simulink subsystem "PowerSystemRef"  (R2024b)
settings: Solver=VariableStepAuto  StartTime=0.0  StopTime=10.0  RelTol=1e-3
undefined symbols (not defined in the file): ess, geom, mot, mot2, mot3, mot4, propel, propel2, propel3, propel4, pxf_diagram_options, SimIn, tc, tc2, tc3, tc4
libraries: simulink x10, slpidlib x5
(part 6 of 10)

== system PowerSystemRef/propel/plant/propel_plant_uas/Thrust_Generated ==
  env_plant_density_simu : Inport
  propel_plant_speed_simu : Inport  Port=2
  Mux5 : Mux  Inputs=3
  RPS2T : Fcn  Expr=u(2) * u(3) * propel.plant.init.propD^4 * u(1)^2
  propel_plant_init_CP_CT_map : Subsystem  mask{x=propel.plant.init.CP_CT_map(:,1)/60, map=propel.plant.init.CP_CT_map(:,2)}
  propel_plant_thrust_simu : Outport  VectorParamsAs1DForOutWhenUnconnected=off
  propel_plant_CT_simu : Outport  Port=2  VectorParamsAs1DForOutWhenUnconnected=off
  wires:
  propel_plant_init_CP_CT_map/1(output) -> propel_plant_CT_simu/1, Mux5/2
  env_plant_density_simu/1 -> Mux5/3
  propel_plant_speed_simu/1 -> propel_plant_init_CP_CT_map/1(input x), Mux5/1
  Mux5/1 -> RPS2T/1
  RPS2T/1 -> propel_plant_thrust_simu/1

== system PowerSystemRef/propel/plant/propel_plant_uas/Total_Moment ==
  propel_plant_thrust_simu : Inport
  propel_plant_restq_simu : Inport  Port=2
  Gain : Gain  Gain=-propel.plant.init.rotationdir
  Gain1 : Gain  Gain=propel.plant.init.thrustdir
  Moment_due_to_eng_position : Subsystem
  Sum2 : Sum  Inputs=|+-  SaturateOnIntegerOverflow=on
  Sum4 : Sum  SaturateOnIntegerOverflow=on
  geom.init.CG : Constant  Value=SimIn.Model.cm_b
  propel.plant.init.pos : Constant  Value=propel.plant.init.pos
  accmoment_plant_totmoment_simu : Outport  VectorParamsAs1DForOutWhenUnconnected=off
  wires:
  propel_plant_restq_simu/1 -> Gain/1
  Gain1/1 -> Moment_due_to_eng_position/2(Vec 2)
  Gain/1 -> Sum4/2
  Sum2/1 -> Moment_due_to_eng_position/1(Vec 1)
  Sum4/1 -> accmoment_plant_totmoment_simu/1  "accmoment_plant_totmoment_simu"
  propel.plant.init.pos/1 -> Sum2/1
  geom.init.CG/1 -> Sum2/2
  propel_plant_thrust_simu/1 -> Gain1/1
  Moment_due_to_eng_position/1(X Prod) -> Sum4/1

== system PowerSystemRef/tc/plant/tc_plant_map_trqloss_funTW/Inertia calculation ==
  inertia in : Inport
  Sum3 : Sum  Inputs=|++  InputSameDT=on  SaturateOnIntegerOverflow=on  OutDataTypeStr=Inherit: Same as first input
  tc inertia : Constant  Value=tc.plant.init.inertia
  tc.plant.init.ratio : Gain  Gain=tc.plant.init.ratio
  "tc.plant.init.ratio " : Gain  Gain=tc.plant.init.ratio
  inertia out : Outport
  wires:
  "tc.plant.init.ratio "/1 -> tc.plant.init.ratio/1
  inertia in/1 -> "tc.plant.init.ratio "/1
  tc.plant.init.ratio/1 -> Sum3/1
  tc inertia/1 -> Sum3/2
  Sum3/1 -> inertia out/1

== system PowerSystemRef/tc/plant/tc_plant_map_trqloss_funTW/Speed calculation ==
  spd out : Inport
  tc.plant.init.ratio : Gain  Gain=tc.plant.init.ratio
  spd in : Outport
  wires:
  spd out/1 -> tc.plant.init.ratio/1
  tc.plant.init.ratio/1 -> spd in/1

== system PowerSystemRef/tc/plant/tc_plant_map_trqloss_funTW/Torque calculation ==
  spd in : Inport
  trq in : Inport  Port=2
  Abs : Abs
  Abs1 : Abs
  Blending (state dependent) : Subsystem  mask(State dependent blending){xl=-tc.plant.init.spd_thresh, yl=-1, xc=0, yc=0, xr=tc.plant.init.spd_thresh, yr=1}
      mask prompts: xl "Left point (x):"; yl "Left point (y):"; xc "Center point (x):"; yc "Center point (y):"; xr "Right point (x):"; yr "Right point (y):"
      mask help: This block implements state dependent smoothing/blending. IMPORTANT: See help menu.
      mask Help: The output equals the product of the first input and a "hat" function defined by the three points specified in the dialog box.  The second input forms the argument to the hat function.\n\nIMPORTANT: A divide by zero error will result if first coordinates of the three points specified for the hat function are NOT distinct.
      mask Display: plot([-1 1 3 6 8], [1.5 1.5 0.5 4.0 4.0])
  Sum2 : Sum  Inputs=|+-  InputSameDT=on  SaturateOnIntegerOverflow=on  OutDataTypeStr=Inherit: Same as first input
  tc.plant.init.ratio : Gain  Gain=tc.plant.init.ratio
  trq losses : Subsystem  mask(Lookup Table (2-D)){x=tc.plant.init.trq_loss.idx1_trq, y=tc.plant.init.trq_loss.idx2_spd, t=tc.plant.init.trq_loss.map}
      mask prompts: x "Row:"; y "Column:"; t "Table:"
      mask help: Performs 2-D linear interpolation of input values using the specified input/output table. Extrapolation is performed outside the table boundaries.
      mask init:
      | [r,c]=size(t);
      | xt=reshape(x,prod(size(x)),1);
      | xi=xt(:,ones(1,c));
      | minx=min(x); maxx=max(x);
      | mint=min(min(t)); maxt=max(max(t));
      mask Display: plot(xi,t,[minx maxx],[mint mint],[minx minx],[mint maxt])
  trq out : Outport
  wires:
  tc.plant.init.ratio/1 -> trq out/1
  Sum2/1 -> tc.plant.init.ratio/1
  trq in/1 -> Sum2/1, Abs/1
  spd in/1 -> Blending (state dependent)/2(Control (state)), Abs1/1
  Blending (state dependent)/1(Output) -> Sum2/2
  trq losses/1(Out1) -> Blending (state dependent)/1(Input)
  Abs1/1 -> trq losses/2(Cols)
  Abs/1 -> trq losses/1(Rows)

== system PowerSystemRef/ess (battery)/ctrl/ess_ctrl_pngv_map_anl_PI_cstr/PI controller for maximal charge power and current1/PI Ratio Calculator (curr)  ==
  note: %deviation
  ess curr : Inport
  curr max cont : Inport  Port=2
  Add1 : Sum  Inputs=-+
  Integrator1 : Integrator  InitialCondition=ess.plant.init.ul_curr_chg  LimitOutput=on  UpperSaturationLimit=ess.plant.init.ul_curr_chg  LowerSaturationLimit=ess.plant.init.ll_curr_chg
  Ki_curr : Gain  Gain=ess.plant.init.Ki_curr_chg  SaturateOnIntegerOverflow=on  OutDataTypeStr=Inherit: Same as input  ParamDataTypeStr=Inherit: Same as input
  Saturation1 : Saturate  UpperLimit=1  LowerLimit=0
  non-zero division1 : Subsystem
      mask Display: disp('divider')
  Current ratio : Outport
  wires:
  Add1/1 -> non-zero division1/1(In1)
  non-zero division1/1(Out1) -> Ki_curr/1
  Ki_curr/1 -> Integrator1/1
  Integrator1/1 -> Saturation1/1
  ess curr/1 -> Add1/1
  Saturation1/1 -> Current ratio/1
  curr max cont/1 -> Add1/2, non-zero division1/2(In2)

== system PowerSystemRef/ess (battery)/ctrl/ess_ctrl_pngv_map_anl_PI_cstr/PI controller for maximal charge power and current1/PI Ratio Calculator (curr) 1 ==
  note: %deviation
  ess pwr : Inport
  pwr max cont : Inport  Port=2
  Add1 : Sum  Inputs=-+
  Integrator1 : Integrator  InitialCondition=ess.plant.init.ul_curr_dis  LimitOutput=on  UpperSaturationLimit=ess.plant.init.ul_curr_dis  LowerSaturationLimit=ess.plant.init.ll_curr_dis
  Ki_pwr : Gain  Gain=ess.plant.init.Ki_pwr_chg  SaturateOnIntegerOverflow=on  OutDataTypeStr=Inherit: Same as input  ParamDataTypeStr=Inherit: Same as input
  Saturation1 : Saturate  UpperLimit=1  LowerLimit=0
  non-zero division1 : Subsystem
      mask Display: disp('divider')
  pwr ratio : Outport
  wires:
  Add1/1 -> non-zero division1/1(In1)
  non-zero division1/1(Out1) -> Ki_pwr/1
  Ki_pwr/1 -> Integrator1/1
  Integrator1/1 -> Saturation1/1
  ess pwr/1 -> Add1/1
  Saturation1/1 -> pwr ratio/1
  pwr max cont/1 -> Add1/2, non-zero division1/2(In2)

== system PowerSystemRef/ess (battery)/ctrl/ess_ctrl_pngv_map_anl_PI_cstr/PI controller for maximal discharge power and current1/PI Ratio Calculator (curr)  ==
  note: %deviation
  ess curr : Inport
  curr max cont : Inport  Port=2
  Add1 : Sum  Inputs=-+
  Integrator1 : Integrator  InitialCondition=ess.plant.init.ul_curr_dis  LimitOutput=on  UpperSaturationLimit=ess.plant.init.ul_curr_dis  LowerSaturationLimit=ess.plant.init.ll_curr_dis
  Ki_curr : Gain  Gain=ess.plant.init.Ki_curr_dis  SaturateOnIntegerOverflow=on  OutDataTypeStr=Inherit: Same as input  ParamDataTypeStr=Inherit: Same as input
  Saturation1 : Saturate  UpperLimit=1  LowerLimit=0
  non-zero division1 : Subsystem
      mask Display: disp('divider')
  Current ratio : Outport
  wires:
  curr max cont/1 -> non-zero division1/2(In2), Add1/2
  Saturation1/1 -> Current ratio/1
  ess curr/1 -> Add1/1
  Integrator1/1 -> Saturation1/1
  Ki_curr/1 -> Integrator1/1
  non-zero division1/1(Out1) -> Ki_curr/1
  Add1/1 -> non-zero division1/1(In1)

== system PowerSystemRef/ess (battery)/ctrl/ess_ctrl_pngv_map_anl_PI_cstr/PI controller for maximal discharge power and current1/PI Ratio Calculator (curr) 1 ==
  note: %deviation
  ess pwr : Inport
  pwr max cont : Inport  Port=2
  Add1 : Sum  Inputs=-+
  Integrator1 : Integrator  InitialCondition=ess.plant.init.ul_curr_dis  LimitOutput=on  UpperSaturationLimit=ess.plant.init.ul_curr_dis  LowerSaturationLimit=ess.plant.init.ll_curr_dis
  Ki_pwr : Gain  Gain=ess.plant.init.Ki_pwr_dis  SaturateOnIntegerOverflow=on  OutDataTypeStr=Inherit: Same as input  ParamDataTypeStr=Inherit: Same as input
  Saturation1 : Saturate  UpperLimit=1  LowerLimit=0
  non-zero division1 : Subsystem
      mask Display: disp('divider')
  pwr ratio : Outport
  wires:
  Add1/1 -> non-zero division1/1(In1)
  non-zero division1/1(Out1) -> Ki_pwr/1
  Ki_pwr/1 -> Integrator1/1
  Integrator1/1 -> Saturation1/1
  ess pwr/1 -> Add1/1
  Saturation1/1 -> pwr ratio/1
  pwr max cont/1 -> Add1/2, non-zero division1/2(In2)

== system PowerSystemRef/ess (battery)/plant/ess_plant_pngv_map_anl_PI_cstr/ess_cell/current polarization ==
  ess soc : Inport
  ess curr : Inport  Port=2
  Integrator : Integrator
  Product1 : Product  Inputs=*/  InputSameDT=on  SaturateOnIntegerOverflow=on  OutDataTypeStr=Inherit: Same as first input
  Sum1 : Sum  Inputs=+-  InputSameDT=on  SaturateOnIntegerOverflow=on  OutDataTypeStr=Inherit: Same as first input
  Time Constant : Lookup  InputValues=ess.plant.init.tau1.idx1_soc  Table=ess.plant.init.tau1.map
  ess_cell_curr_polar1 : Outport
  wires:
  Time Constant/1 -> Product1/2
  Product1/1 -> Integrator/1
  ess soc/1 -> Time Constant/1
  ess curr/1 -> Sum1/1
  Sum1/1 -> Product1/1
  Integrator/1 -> Sum1/2, ess_cell_curr_polar1/1

== system PowerSystemRef/ess (battery)/plant/ess_plant_pngv_map_anl_PI_cstr/ess_cell/current polarization1 ==
  ess soc : Inport
  ess curr : Inport  Port=2
  Integrator : Integrator
  Product1 : Product  Inputs=*/  InputSameDT=on  SaturateOnIntegerOverflow=on  OutDataTypeStr=Inherit: Same as first input
  Sum1 : Sum  Inputs=+-  InputSameDT=on  SaturateOnIntegerOverflow=on  OutDataTypeStr=Inherit: Same as first input
  Time Constant : Lookup  InputValues=ess.plant.init.tau2.idx1_soc  Table=ess.plant.init.tau2.map
  ess_cell_curr_polar2 : Outport
  wires:
  Integrator/1 -> ess_cell_curr_polar2/1, Sum1/2
  Sum1/1 -> Product1/1
  ess curr/1 -> Sum1/1
  ess soc/1 -> Time Constant/1
  Product1/1 -> Integrator/1
  Time Constant/1 -> Product1/2

== system PowerSystemRef/ess (battery)/plant/ess_plant_pngv_map_anl_PI_cstr/ess_cell/ess_soc_calculation ==
  cell_curr : Inport
  (sec->hrs) : Gain  Gain=1/3600  SaturateOnIntegerOverflow=on  OutDataTypeStr=Inherit: Same as input  ParamDataTypeStr=Inherit: Same as input
  (sec->hrs)1 : Gain  Gain=-1  SaturateOnIntegerOverflow=on  OutDataTypeStr=Inherit: Same as input  ParamDataTypeStr=Inherit: Same as input
  0 <= SOC <= 1 : Saturate  UpperLimit=1  LowerLimit=0
  1\ess.plant.init.cap : Gain  Gain=1/ess.plant.init.cap  SaturateOnIntegerOverflow=on  OutDataTypeStr=Inherit: Same as input  ParamDataTypeStr=Inherit: Same as input
  Integrator : Integrator  InitialCondition=ess.plant.init.soc_init
  ess_soc : Outport
  wires:
  (sec->hrs)/1 -> 1\ess.plant.init.cap/1
  0 <= SOC <= 1/1 -> ess_soc/1
  Integrator/1 -> 0 <= SOC <= 1/1
  (sec->hrs)1/1 -> Integrator/1
  1\ess.plant.init.cap/1 -> (sec->hrs)1/1
  cell_curr/1 -> (sec->hrs)/1

== system PowerSystemRef/ess (battery)/plant/ess_plant_pngv_map_anl_PI_cstr/ess_cell/voltage calculation ==
  absolute SOC : Inport
  ess_cell_curr : Inport  Port=2
  ess_cell_curr_pol1 : Inport  Port=3
  ess_cell_curr_plo2 : Inport  Port=4
  Ohmic resist : Lookup  InputValues=ess.plant.init.rint.idx1_soc  Table=ess.plant.init.rint.map
  "Polarization resist 2 " : Lookup  InputValues=ess.plant.init.rpol2.idx1_soc  Table=ess.plant.init.rpol2.map
  Polarization resist2 : Lookup  InputValues=ess.plant.init.rpol1.idx1_soc  Table=ess.plant.init.rpol1.map
  Product1 : Product  InputSameDT=on  SaturateOnIntegerOverflow=on  OutDataTypeStr=Inherit: Same as first input
  Product2 : Product  InputSameDT=on  SaturateOnIntegerOverflow=on  OutDataTypeStr=Inherit: Same as first input
  Product3 : Product  InputSameDT=on  SaturateOnIntegerOverflow=on  OutDataTypeStr=Inherit: Same as first input
  Saturation : Saturate  UpperLimit=inf  LowerLimit=ess.plant.init.volt_min_burst
  Sum2 : Sum  Inputs=+---  InputSameDT=on  SaturateOnIntegerOverflow=on  OutDataTypeStr=Inherit: Same as first input
  Voc : Lookup  InputValues=ess.plant.init.voc.idx1_soc  Table=ess.plant.init.voc.map
  ess_cell_volt : Outport
  ess_cell_voc : Outport  Port=2
  ess_cell_rint : Outport  Port=3
  ess_cell_rpol1 : Outport  Port=4
  ess_cell_rpol2 : Outport  Port=5
  wires:
  Saturation/1 -> ess_cell_volt/1
  "Polarization resist 2 "/1 -> ess_cell_rpol2/1, Product3/2  "ess_rpol2_simu"
  ess_cell_curr_plo2/1 -> Product3/1
  Product3/1 -> Sum2/4
  Product2/1 -> Sum2/3
  Polarization resist2/1 -> ess_cell_rpol1/1, Product2/2  "ess_rpol1_simu"
  ess_cell_curr_pol1/1 -> Product2/1
  Product1/1 -> Sum2/2
  absolute SOC/1 -> Voc/1, Ohmic resist/1, Polarization resist2/1, "Polarization resist 2 "/1
  Voc/1 -> ess_cell_voc/1, Sum2/1  "ess_voc_simu"
  ess_cell_curr/1 -> Product1/1
  Ohmic resist/1 -> ess_cell_rint/1, Product1/2  "ess_rint_simu"
  Sum2/1 -> Saturation/1

== system PowerSystemRef/mot/ctrl/cmd/mot_ctrl_cmd_map_Pelec_funTW_volt_in/Subsystem2 ==
  In1 : Inport
  In2 : Inport  Port=2
  Fcn : Fcn  Expr=u[1]/(u[2]+eps)*(u[2]!=0)
  Mux : Mux  Inputs=2
  Out1 : Outport
  wires:
  In2/1 -> Mux/2
  Fcn/1 -> Out1/1
  In1/1 -> Mux/1
  Mux/1 -> Fcn/1

== system PowerSystemRef/mot/ctrl/cmd/mot_ctrl_cmd_map_Pelec_funTW_volt_in/avoid zero output ==
  In1 : Inport
  Constant : Constant  Value=eps
  Switch1 : Switch  Criteria=u2 ~= 0  SaturateOnIntegerOverflow=off  InputSameDT=off
  Out1 : Outport
  wires:
  In1/1 -> Switch1/2, Switch1/1
  Constant/1 -> Switch1/3
  Switch1/1 -> Out1/1

== system PowerSystemRef/mot/ctrl/cstr/mot_ctrl_cstr_map_Pelec_funTW_volt_in/Continuous torque - Prop ==
  input x : Inport
  map : Lookup  InputValues=x  Table=map
  map limits on x : Saturate  UpperLimit=max(x)  LowerLimit=min(x)
  output : Outport
  wires:
  map limits on x/1 -> map/1
  map/1 -> output/1
  input x/1 -> map limits on x/1

== system PowerSystemRef/mot/ctrl/cstr/mot_ctrl_cstr_map_Pelec_funTW_volt_in/Continuous torque _regen ==
  input x : Inport
  map : Lookup  InputValues=x  Table=map
  map limits on x : Saturate  UpperLimit=max(x)  LowerLimit=min(x)
  output : Outport
  wires:
  map limits on x/1 -> map/1
  map/1 -> output/1
  input x/1 -> map limits on x/1

== system PowerSystemRef/mot/ctrl/cstr/mot_ctrl_cstr_map_Pelec_funTW_volt_in/Peak torque - Prop ==
  input x : Inport
  map : Lookup  InputValues=x  Table=map
  map limits on x : Saturate  UpperLimit=max(x)  LowerLimit=min(x)
  output : Outport
  wires:
  map limits on x/1 -> map/1
  map/1 -> output/1
  input x/1 -> map limits on x/1

== system PowerSystemRef/mot/ctrl/cstr/mot_ctrl_cstr_map_Pelec_funTW_volt_in/Peak torque _regen ==
  input x : Inport
  map : Lookup  InputValues=x  Table=map
  map limits on x : Saturate  UpperLimit=max(x)  LowerLimit=min(x)
  output : Outport
  wires:
  map limits on x/1 -> map/1
  map/1 -> output/1
  input x/1 -> map limits on x/1

== system PowerSystemRef/mot/ctrl/dmd/mot_ctrl_dmd_uas/Determine_Required_Motor_RPS ==
  Prop_D : Inport
  rho : Inport  Port=2
  P : Inport  Port=3
  CPpoly : Inport  Port=4
  Algebraic Constraint : AlgebraicConstraint  InitialGuess=100
  Demux : Demux  Outputs=2
  Fcn : Fcn  Expr=u(4)*u(6)^4 + u(5)*u(6)^3 - u(3)/u(2)/u(1)^5
  MATLAB Function : MATLAB Function  Commented=on  TreatAsAtomicUnit=on
  Mux : Mux  Inputs=6
  RPS_req : Outport  VectorParamsAs1DForOutWhenUnconnected=off
  wires:
  Fcn/1 -> Algebraic Constraint/1
  Algebraic Constraint/1 -> Mux/6, RPS_req/1  "RPS_req"
  Mux/1 -> Fcn/1
  CPpoly/1 -> Demux/1
  Demux/2 -> Mux/5
  Demux/1 -> Mux/4
  Prop_D/1 -> Mux/1
  P/1 -> Mux/3
  rho/1 -> Mux/2

== system PowerSystemRef/mot/ctrl/dmd/mot_ctrl_dmd_uas/mot_propel_plant_init_eff_map ==
  input x : Inport
  map : Lookup  InputValues=x  Table=map
  map limits on x : Saturate  UpperLimit=max(x)  LowerLimit=min(x)
  output : Outport  VectorParamsAs1DForOutWhenUnconnected=off
  wires:
  input x/1 -> map limits on x/1
  map/1 -> output/1
  map limits on x/1 -> map/1

== system PowerSystemRef/mot/plant/mot_plant_map_Pelec_funTW_volt_in/max torque /Cont trq max - Prop ==
  input x : Inport
  map : Lookup  InputValues=x  Table=map
  map limits on x : Saturate  UpperLimit=max(x)  LowerLimit=min(x)
  output : Outport
  wires:
  input x/1 -> map limits on x/1
  map/1 -> output/1
  map limits on x/1 -> map/1

== system PowerSystemRef/mot/plant/mot_plant_map_Pelec_funTW_volt_in/max torque /Cont trq max - Regen ==
  input x : Inport
  map : Lookup  InputValues=x  Table=map
  map limits on x : Saturate  UpperLimit=max(x)  LowerLimit=min(x)
  output : Outport
  wires:
  map limits on x/1 -> map/1
  map/1 -> output/1
  input x/1 -> map limits on x/1

== system PowerSystemRef/mot/plant/mot_plant_map_Pelec_funTW_volt_in/max torque /Heat index ==
  note: Heat index calculation
  note: to avoid spikes
      |  due to
      | div by zero
  cont torque : Inport
  torque : Inport  Port=2
  Abs : Abs
  Divide : Subsystem  mask(Divide){}
      mask Display: disp('Divide')
  Heat Energy Factor : Integrator  InitialCondition=-0.3  LimitOutput=on  UpperSaturationLimit=1  LowerSaturationLimit=-0.3
  Heating Constant : Gain  Gain=0.3/mot.plant.init.t_max_trq  SaturateOnIntegerOverflow=on  OutDataTypeStr=Inherit: Same as input  ParamDataTypeStr=Inherit: Same as input
  Saturation : Saturate  UpperLimit=1  LowerLimit=0
  Saturation1 : Saturate  UpperLimit=10  LowerLimit=0
  Sum : Sum  Inputs=+-  InputSameDT=on  SaturateOnIntegerOverflow=on  OutDataTypeStr=Inherit: Same as first input
  motor inertia (Nms^2\rad)5 : Constant
  Heat index : Outport
  wires:
  Saturation1/1 -> Sum/1
  torque/1 -> Divide/1(numerator)
  Heat Energy Factor/1 -> Saturation/1
  Heating Constant/1 -> Heat Energy Factor/1
  Sum/1 -> Heating Constant/1
  Divide/1(quotient) -> Abs/1
  motor inertia (Nms^2\rad)5/1 -> Sum/2
  Saturation/1 -> Heat index/1
  Abs/1 -> Saturation1/1
  cont torque/1 -> Divide/2(denominator)

== system PowerSystemRef/mot/plant/mot_plant_map_Pelec_funTW_volt_in/max torque /Peak trq max - Prop ==
  input x : Inport
  map : Lookup  InputValues=x  Table=map
  map limits on x : Saturate  UpperLimit=max(x)  LowerLimit=min(x)
  output : Outport
  wires:
  map limits on x/1 -> map/1
  map/1 -> output/1
  input x/1 -> map limits on x/1

== system PowerSystemRef/mot/plant/mot_plant_map_Pelec_funTW_volt_in/max torque /Peak trq max - Regen ==
  input x : Inport
  map : Lookup  InputValues=x  Table=map
  map limits on x : Saturate  UpperLimit=max(x)  LowerLimit=min(x)
  output : Outport
  wires:
  input x/1 -> map limits on x/1
  map/1 -> output/1
  map limits on x/1 -> map/1

== system PowerSystemRef/powerplant/ess (battery)/ctrl/ess_ctrl_pngv_map_anl_PI_cstr/PI controller for maximal charge power and current1 ==
  ess voltage : Inport
  ess curr : Inport  Port=2
  SOC : Inport  Port=3
  Burst maximal power : Lookup  InputValues=ess.plant.init.pwr_chg_10sec.idx1_soc  Table=ess.plant.init.pwr_chg_10sec.map  SaturateOnIntegerOverflow=off
  Continuous maximal power : Lookup  InputValues=ess.plant.init.pwr_chg.idx1_soc  Table=ess.plant.init.pwr_chg.map  SaturateOnIntegerOverflow=off
  Interpolation (curr) : Fcn  Expr=u(3)*u(1) + u(2)*(1-u(1))
  Interpolation (curr)1 : Fcn  Expr=u(3)*u(1) + u(2)*(1-u(1))
  Mux1 : Mux  Inputs=3
  Mux2 : Mux  Inputs=3
  "PI Ratio Calculator (curr) " : Subsystem
  PI Ratio Calculator (curr) 1 : Subsystem
  Product : Product  RndMeth=Zero
  Saturation : Saturate  UpperLimit=0  LowerLimit=-inf
  Saturation1 : Saturate  UpperLimit=0  LowerLimit=-inf
  "ess curr " : InportShadow  Port=2
  ess maximum current (burst charge) : Lookup  InputValues=ess.plant.init.curr_chg_burst_max.idx1_soc  Table=ess.plant.init.curr_chg_burst_max.map  SaturateOnIntegerOverflow=off
  ess maximum current (continuous charge) : Lookup  InputValues=ess.plant.init.curr_chg_cont_max.idx1_soc  Table=ess.plant.init.curr_chg_cont_max.map  SaturateOnIntegerOverflow=off
  ess.init.num_cell1 : Gain  Gain=ess.plant.init.num_cell  SaturateOnIntegerOverflow=on  OutDataTypeStr=Inherit: Same as input  ParamDataTypeStr=Inherit: Same as input
  ess.init.num_cell2 : Gain  Gain=ess.plant.init.num_cell  SaturateOnIntegerOverflow=on  OutDataTypeStr=Inherit: Same as input  ParamDataTypeStr=Inherit: Same as input
  ess.init.num_module_parallel1 : Gain  Gain=ess.plant.init.num_module_parallel
  ess.init.num_module_parallel5 : Gain  Gain=ess.plant.init.num_module_parallel
  Pwr_max_reg : Outport
  Curr_max_reg : Outport  Port=2
  wires:
  ess.init.num_module_parallel1/1 -> Mux1/3
  ess.init.num_module_parallel5/1 -> "PI Ratio Calculator (curr) "/2(curr max cont), Mux1/2
  ess.init.num_cell1/1 -> Mux2/3
  ess.init.num_cell2/1 -> PI Ratio Calculator (curr) 1/2(pwr max cont), Mux2/2
  Product/1 -> Saturation1/1
  ess voltage/1 -> Product/1
  "ess curr "/1 -> Product/2
  Burst maximal power/1 -> ess.init.num_cell1/1
  PI Ratio Calculator (curr) 1/1(pwr ratio) -> Mux2/1
  Mux2/1 -> Interpolation (curr)1/1
  Interpolation (curr)1/1 -> Pwr_max_reg/1
  Continuous maximal power/1 -> ess.init.num_cell2/1
  Saturation1/1 -> PI Ratio Calculator (curr) 1/1(ess pwr)
  SOC/1 -> ess maximum current (burst charge)/1, ess maximum current (continuous charge)/1, Burst maximal power/1, Continuous maximal power/1
  Interpolation (curr)/1 -> Curr_max_reg/1
  Mux1/1 -> Interpolation (curr)/1
  ess curr/1 -> Saturation/1
  ess maximum current (continuous charge)/1 -> ess.init.num_module_parallel5/1
  ess maximum current (burst charge)/1 -> ess.init.num_module_parallel1/1
  "PI Ratio Calculator (curr) "/1(Current ratio) -> Mux1/1
  Saturation/1 -> "PI Ratio Calculator (curr) "/1(ess curr)

== system PowerSystemRef/powerplant/ess (battery)/ctrl/ess_ctrl_pngv_map_anl_PI_cstr/PI controller for maximal discharge power and current1 ==
  ess voltage : Inport
  ess curr : Inport  Port=2
  SOC : Inport  Port=3
  Burst maximal power : Lookup  InputValues=ess.plant.init.pwr_dis_10sec.idx1_soc  Table=ess.plant.init.pwr_dis_10sec.map  SaturateOnIntegerOverflow=off
  Continuous maximal power : Lookup  InputValues=ess.plant.init.pwr_dis.idx1_soc  Table=ess.plant.init.pwr_dis.map  SaturateOnIntegerOverflow=off
  Interpolation (curr) : Fcn  Expr=u(3)*u(1) + u(2)*(1-u(1))
  Interpolation (curr)1 : Fcn  Expr=u(3)*u(1) + u(2)*(1-u(1))
  Mux1 : Mux  Inputs=3
  Mux2 : Mux  Inputs=3
  "PI Ratio Calculator (curr) " : Subsystem
  PI Ratio Calculator (curr) 1 : Subsystem
  Product : Product  RndMeth=Zero
  Saturation : Saturate  UpperLimit=inf  LowerLimit=0
  Saturation1 : Saturate  UpperLimit=inf  LowerLimit=0
  "ess curr " : InportShadow  Port=2
  ess maximum current (burst discharge)1 : Lookup  InputValues=ess.plant.init.curr_dis_burst_max.idx1_soc  Table=ess.plant.init.curr_dis_burst_max.map  SaturateOnIntegerOverflow=off
  "ess maximum current (continuous discharge) " : Lookup  InputValues=ess.plant.init.curr_dis_cont_max.idx1_soc  Table=ess.plant.init.curr_dis_cont_max.map  SaturateOnIntegerOverflow=off
  ess.init.num_cell1 : Gain  Gain=ess.plant.init.num_cell  SaturateOnIntegerOverflow=on  OutDataTypeStr=Inherit: Same as input  ParamDataTypeStr=Inherit: Same as input
  ess.init.num_cell2 : Gain  Gain=ess.plant.init.num_cell  SaturateOnIntegerOverflow=on  OutDataTypeStr=Inherit: Same as input  ParamDataTypeStr=Inherit: Same as input
  ess.init.num_module_parallel1 : Gain  Gain=ess.plant.init.num_module_parallel
  ess.init.num_module_parallel5 : Gain  Gain=ess.plant.init.num_module_parallel
  Curr_max_prop : Outport
  Pwr_max_prop : Outport  Port=2
  wires:
  ess.init.num_module_parallel1/1 -> Mux1/3
  ess.init.num_module_parallel5/1 -> Mux1/2, "PI Ratio Calculator (curr) "/2(curr max cont)
  ess.init.num_cell2/1 -> Mux2/3
  ess.init.num_cell1/1 -> PI Ratio Calculator (curr) 1/2(pwr max cont), Mux2/2
  Product/1 -> Saturation1/1
  ess voltage/1 -> Product/1
  "ess curr "/1 -> Product/2
  Burst maximal power/1 -> ess.init.num_cell2/1
  PI Ratio Calculator (curr) 1/1(pwr ratio) -> Mux2/1
  Mux2/1 -> Interpolation (curr)1/1
  Interpolation (curr)1/1 -> Pwr_max_prop/1
  Continuous maximal power/1 -> ess.init.num_cell1/1
  Saturation1/1 -> PI Ratio Calculator (curr) 1/1(ess pwr)
  SOC/1 -> ess maximum current (burst discharge)1/1, "ess maximum current (continuous discharge) "/1, Burst maximal power/1, Continuous maximal power/1
  Saturation/1 -> "PI Ratio Calculator (curr) "/1(ess curr)
  "PI Ratio Calculator (curr) "/1(Current ratio) -> Mux1/1
  ess maximum current (burst discharge)1/1 -> ess.init.num_module_parallel1/1
  "ess maximum current (continuous discharge) "/1 -> ess.init.num_module_parallel5/1
  ess curr/1 -> Saturation/1
  Mux1/1 -> Interpolation (curr)/1
  Interpolation (curr)/1 -> Curr_max_prop/1

== system PowerSystemRef/powerplant/ess (battery)/plant/ess_plant_pngv_map_anl_PI_cstr/ess_cell ==
  ess_cell_curr : Inport
  Memory : Memory
  current polarization : Subsystem
  current polarization1 : Subsystem
  ess_soc_calculation : Subsystem
  voltage calculation : Subsystem
  ess_cell_volt_out : Outport
  ess_cell_soc : Outport  Port=2
  ess_cell_voc : Outport  Port=3
  ess_cell_rint : Outport  Port=4
  ess_cell_rpol1 : Outport  Port=5
  ess_cell_rpol2 : Outport  Port=6
  ess_cell_curr_polar2 : Outport  Port=7
  ess_cell_curr_polar1 : Outport  Port=8
  wires:
  ess_cell_curr/1 -> Memory/1
  voltage calculation/5(ess_cell_rpol2) -> ess_cell_rpol2/1
  voltage calculation/4(ess_cell_rpol1) -> ess_cell_rpol1/1
  voltage calculation/3(ess_cell_rint) -> ess_cell_rint/1
  voltage calculation/2(ess_cell_voc) -> ess_cell_voc/1
  voltage calculation/1(ess_cell_volt) -> ess_cell_volt_out/1
  current polarization1/1(ess_cell_curr_polar2) -> voltage calculation/4(ess_cell_curr_plo2), ess_cell_curr_polar2/1
  ess_soc_calculation/1(ess_soc) -> current polarization1/1(ess soc), voltage calculation/1(absolute SOC), ess_cell_soc/1, current polarization/1(ess soc)
  Memory/1 -> ess_soc_calculation/1(cell_curr), current polarization1/2(ess curr), current polarization/2(ess curr), voltage calculation/2(ess_cell_curr)
  current polarization/1(ess_cell_curr_polar1) -> voltage calculation/3(ess_cell_curr_pol1), ess_cell_curr_polar1/1

== system PowerSystemRef/powerplant/ess (battery)/plant/ess_plant_pngv_map_anl_PI_cstr/heat_generated ==
  volt_out : Inport
  ocv : Inport  Port=2
  load_current : Inport  Port=3
  Add : Sum  Inputs=-+
  Divide : Product  Inputs=*/
  Memory : Memory  InitialCondition=eps
  Product : Product  RndMeth=Zero
  square : Math  Operator=square  SignedPower=on
  heat_J : Outport
  impedance : Outport  Port=2
  wires:
  Memory/1 -> Divide/2, square/1
  Divide/1 -> impedance/1, Product/1  "R"
  Add/1 -> Divide/1
  Product/1 -> heat_J/1
  square/1 -> Product/2  "I sq"
  load_current/1 -> Memory/1
  ocv/1 -> Add/2
  volt_out/1 -> Add/1

== system PowerSystemRef/powerplant/ess (battery)1/ctrl/ess_ctrl_pngv_map_anl_PI_cstr/PI controller for maximal charge power and current1 ==
  ess voltage : Inport
  ess curr : Inport  Port=2
  SOC : Inport  Port=3
  Burst maximal power : Lookup  InputValues=ess.plant.init.pwr_chg_10sec.idx1_soc  Table=ess.plant.init.pwr_chg_10sec.map  SaturateOnIntegerOverflow=off
  Continuous maximal power : Lookup  InputValues=ess.plant.init.pwr_chg.idx1_soc  Table=ess.plant.init.pwr_chg.map  SaturateOnIntegerOverflow=off
  Interpolation (curr) : Fcn  Expr=u(3)*u(1) + u(2)*(1-u(1))
  Interpolation (curr)1 : Fcn  Expr=u(3)*u(1) + u(2)*(1-u(1))
  Mux1 : Mux  Inputs=3
  Mux2 : Mux  Inputs=3
  "PI Ratio Calculator (curr) " : Subsystem
  PI Ratio Calculator (curr) 1 : Subsystem
  Product : Product  RndMeth=Zero
  Saturation : Saturate  UpperLimit=0  LowerLimit=-inf
  Saturation1 : Saturate  UpperLimit=0  LowerLimit=-inf
  "ess curr " : InportShadow  Port=2
  ess maximum current (burst charge) : Lookup  InputValues=ess.plant.init.curr_chg_burst_max.idx1_soc  Table=ess.plant.init.curr_chg_burst_max.map  SaturateOnIntegerOverflow=off
  ess maximum current (continuous charge) : Lookup  InputValues=ess.plant.init.curr_chg_cont_max.idx1_soc  Table=ess.plant.init.curr_chg_cont_max.map  SaturateOnIntegerOverflow=off
  ess.init.num_cell1 : Gain  Gain=ess.plant.init.num_cell  SaturateOnIntegerOverflow=on  OutDataTypeStr=Inherit: Same as input  ParamDataTypeStr=Inherit: Same as input
  ess.init.num_cell2 : Gain  Gain=ess.plant.init.num_cell  SaturateOnIntegerOverflow=on  OutDataTypeStr=Inherit: Same as input  ParamDataTypeStr=Inherit: Same as input
  ess.init.num_module_parallel1 : Gain  Gain=ess.plant.init.num_module_parallel
  ess.init.num_module_parallel5 : Gain  Gain=ess.plant.init.num_module_parallel
  Pwr_max_reg : Outport
  Curr_max_reg : Outport  Port=2
  wires:
  Saturation/1 -> "PI Ratio Calculator (curr) "/1(ess curr)
  "PI Ratio Calculator (curr) "/1(Current ratio) -> Mux1/1
  ess maximum current (burst charge)/1 -> ess.init.num_module_parallel1/1
  ess maximum current (continuous charge)/1 -> ess.init.num_module_parallel5/1
  ess curr/1 -> Saturation/1
  Mux1/1 -> Interpolation (curr)/1
  Interpolation (curr)/1 -> Curr_max_reg/1
  SOC/1 -> Continuous maximal power/1, Burst maximal power/1, ess maximum current (continuous charge)/1, ess maximum current (burst charge)/1
  Saturation1/1 -> PI Ratio Calculator (curr) 1/1(ess pwr)
  Continuous maximal power/1 -> ess.init.num_cell2/1
  Interpolation (curr)1/1 -> Pwr_max_reg/1
  Mux2/1 -> Interpolation (curr)1/1
  PI Ratio Calculator (curr) 1/1(pwr ratio) -> Mux2/1
  Burst maximal power/1 -> ess.init.num_cell1/1
  "ess curr "/1 -> Product/2
  ess voltage/1 -> Product/1
  Product/1 -> Saturation1/1
  ess.init.num_cell2/1 -> Mux2/2, PI Ratio Calculator (curr) 1/2(pwr max cont)
  ess.init.num_cell1/1 -> Mux2/3
  ess.init.num_module_parallel5/1 -> Mux1/2, "PI Ratio Calculator (curr) "/2(curr max cont)
  ess.init.num_module_parallel1/1 -> Mux1/3

== system PowerSystemRef/powerplant/ess (battery)1/ctrl/ess_ctrl_pngv_map_anl_PI_cstr/PI controller for maximal discharge power and current1 ==
  ess voltage : Inport
  ess curr : Inport  Port=2
  SOC : Inport  Port=3
  Burst maximal power : Lookup  InputValues=ess.plant.init.pwr_dis_10sec.idx1_soc  Table=ess.plant.init.pwr_dis_10sec.map  SaturateOnIntegerOverflow=off
  Continuous maximal power : Lookup  InputValues=ess.plant.init.pwr_dis.idx1_soc  Table=ess.plant.init.pwr_dis.map  SaturateOnIntegerOverflow=off
  Interpolation (curr) : Fcn  Expr=u(3)*u(1) + u(2)*(1-u(1))
  Interpolation (curr)1 : Fcn  Expr=u(3)*u(1) + u(2)*(1-u(1))
  Mux1 : Mux  Inputs=3
  Mux2 : Mux  Inputs=3
  "PI Ratio Calculator (curr) " : Subsystem
  PI Ratio Calculator (curr) 1 : Subsystem
  Product : Product  RndMeth=Zero
  Saturation : Saturate  UpperLimit=inf  LowerLimit=0
  Saturation1 : Saturate  UpperLimit=inf  LowerLimit=0
  "ess curr " : InportShadow  Port=2
  ess maximum current (burst discharge)1 : Lookup  InputValues=ess.plant.init.curr_dis_burst_max.idx1_soc  Table=ess.plant.init.curr_dis_burst_max.map  SaturateOnIntegerOverflow=off
  "ess maximum current (continuous discharge) " : Lookup  InputValues=ess.plant.init.curr_dis_cont_max.idx1_soc  Table=ess.plant.init.curr_dis_cont_max.map  SaturateOnIntegerOverflow=off
  ess.init.num_cell1 : Gain  Gain=ess.plant.init.num_cell  SaturateOnIntegerOverflow=on  OutDataTypeStr=Inherit: Same as input  ParamDataTypeStr=Inherit: Same as input
  ess.init.num_cell2 : Gain  Gain=ess.plant.init.num_cell  SaturateOnIntegerOverflow=on  OutDataTypeStr=Inherit: Same as input  ParamDataTypeStr=Inherit: Same as input
  ess.init.num_module_parallel1 : Gain  Gain=ess.plant.init.num_module_parallel
  ess.init.num_module_parallel5 : Gain  Gain=ess.plant.init.num_module_parallel
  Curr_max_prop : Outport
  Pwr_max_prop : Outport  Port=2
  wires:
  Interpolation (curr)/1 -> Curr_max_prop/1
  Mux1/1 -> Interpolation (curr)/1
  ess curr/1 -> Saturation/1
  "ess maximum current (continuous discharge) "/1 -> ess.init.num_module_parallel5/1
  ess maximum current (burst discharge)1/1 -> ess.init.num_module_parallel1/1
  "PI Ratio Calculator (curr) "/1(Current ratio) -> Mux1/1
  Saturation/1 -> "PI Ratio Calculator (curr) "/1(ess curr)
  SOC/1 -> Continuous maximal power/1, Burst maximal power/1, "ess maximum current (continuous discharge) "/1, ess maximum current (burst discharge)1/1
  Saturation1/1 -> PI Ratio Calculator (curr) 1/1(ess pwr)
  Continuous maximal power/1 -> ess.init.num_cell1/1
  Interpolation (curr)1/1 -> Pwr_max_prop/1
  Mux2/1 -> Interpolation (curr)1/1
  PI Ratio Calculator (curr) 1/1(pwr ratio) -> Mux2/1
  Burst maximal power/1 -> ess.init.num_cell2/1
  "ess curr "/1 -> Product/2
  ess voltage/1 -> Product/1
  Product/1 -> Saturation1/1
  ess.init.num_cell1/1 -> Mux2/2, PI Ratio Calculator (curr) 1/2(pwr max cont)
  ess.init.num_cell2/1 -> Mux2/3
  ess.init.num_module_parallel5/1 -> "PI Ratio Calculator (curr) "/2(curr max cont), Mux1/2
  ess.init.num_module_parallel1/1 -> Mux1/3

== system PowerSystemRef/powerplant/ess (battery)1/plant/ess_plant_pngv_map_anl_PI_cstr/ess_cell ==
  ess_cell_curr : Inport
  Memory : Memory
  current polarization : Subsystem
  current polarization1 : Subsystem
  ess_soc_calculation : Subsystem
  voltage calculation : Subsystem
  ess_cell_volt_out : Outport
  ess_cell_soc : Outport  Port=2
  ess_cell_voc : Outport  Port=3
  ess_cell_rint : Outport  Port=4
  ess_cell_rpol1 : Outport  Port=5
  ess_cell_rpol2 : Outport  Port=6
  ess_cell_curr_polar2 : Outport  Port=7
  ess_cell_curr_polar1 : Outport  Port=8
  wires:
  current polarization/1(ess_cell_curr_polar1) -> ess_cell_curr_polar1/1, voltage calculation/3(ess_cell_curr_pol1)
  Memory/1 -> voltage calculation/2(ess_cell_curr), current polarization/2(ess curr), current polarization1/2(ess curr), ess_soc_calculation/1(cell_curr)
  ess_soc_calculation/1(ess_soc) -> current polarization/1(ess soc), ess_cell_soc/1, voltage calculation/1(absolute SOC), current polarization1/1(ess soc)
  current polarization1/1(ess_cell_curr_polar2) -> ess_cell_curr_polar2/1, voltage calculation/4(ess_cell_curr_plo2)
  voltage calculation/1(ess_cell_volt) -> ess_cell_volt_out/1
  voltage calculation/2(ess_cell_voc) -> ess_cell_voc/1
  voltage calculation/3(ess_cell_rint) -> ess_cell_rint/1
  voltage calculation/4(ess_cell_rpol1) -> ess_cell_rpol1/1
  voltage calculation/5(ess_cell_rpol2) -> ess_cell_rpol2/1
  ess_cell_curr/1 -> Memory/1

== system PowerSystemRef/powerplant/ess (battery)1/plant/ess_plant_pngv_map_anl_PI_cstr/heat_generated ==
  volt_out : Inport
  ocv : Inport  Port=2
  load_current : Inport  Port=3
  Add : Sum  Inputs=-+
  Divide : Product  Inputs=*/
  Memory : Memory  InitialCondition=eps
  Product : Product  RndMeth=Zero
  square : Math  Operator=square  SignedPower=on
  heat_J : Outport
  impedance : Outport  Port=2
  wires:
  volt_out/1 -> Add/1
  ocv/1 -> Add/2
  load_current/1 -> Memory/1
  square/1 -> Product/2  "I sq"
  Product/1 -> heat_J/1
  Add/1 -> Divide/1
  Divide/1 -> Product/1, impedance/1  "R"
  Memory/1 -> square/1, Divide/2

== system PowerSystemRef/powerplant/mot/ctrl/cmd/mot_ctrl_cmd_map_Pelec_funTW_volt_in ==
  mot_plant_spd_out_simu : Inport
  mot_ctrl_trs_trq_simu : Inport  Port=2
  mot_ctrl_cstr_trq_max_pos_simu : Inport  Port=3
  mot_ctrl_cstr_trq_max_neg_simu : Inport  Port=4
  Abs : Abs
  Abs1 : Abs
  Abs2 : Abs
  Fcn : Fcn  Expr=(u>=0) - (u<0)
  Product : Product  SaturateOnIntegerOverflow=on  OutDataTypeStr=Inherit: Same as first input
  Product1 : Product  SaturateOnIntegerOverflow=on  OutDataTypeStr=Inherit: Same as first input
  Subsystem2 : Subsystem
      mask Display: disp('divider')
  Switch : Switch  InputSameDT=off
  "[-1, 1]" : Saturate  UpperLimit=1  LowerLimit=-1
  avoid zero output : Subsystem
  mot_ctrl_cmd_simu : Outport
  wires:
  avoid zero output/1(Out1) -> Product/2
  [mot_ctrl_cmd_simu] -> mot_ctrl_cmd_simu/1  "mot_ctrl_cmd_simu"
  Product1/1 -> [mot_ctrl_cmd_simu]
  mot_ctrl_cstr_trq_max_pos_simu/1 -> Abs1/1
  mot_ctrl_cstr_trq_max_neg_simu/1 -> Abs2/1
  mot_plant_spd_out_simu/1 -> avoid zero output/1(In1)
  Product/1 -> Switch/2, Fcn/1
  Switch/1 -> Subsystem2/2(In2)
  Subsystem2/1(Out1) -> "[-1, 1]"/1
  mot_ctrl_trs_trq_simu/1 -> Product/1, Abs/1
  Abs/1 -> Subsystem2/1(In1)
  Abs1/1 -> Switch/1
  Abs2/1 -> Switch/3
  "[-1, 1]"/1 -> Product1/2
  Fcn/1 -> Product1/1

== system PowerSystemRef/powerplant/mot/ctrl/cmd/parameter_out ==
  inport-mot_ctrl_cmd_simu : Inport
  Toworkspace-mot_ctrl_cmd_simu : ToWorkspace  VariableName=mot_ctrl_cmd_simu  SampleTime=pxf_diagram_options.workspace_sample_time
      settings: Decimation=pxf_diagram_options.decimation
  create_system_info_bus : BusCreator  Inputs=1
  outport-system_info_bus : Outport
  wires:
  create_system_info_bus/1 -> outport-system_info_bus/1
  inport-mot_ctrl_cmd_simu/1 -> create_system_info_bus/1, Toworkspace-mot_ctrl_cmd_simu/1  "mot_ctrl_cmd_simu"

== system PowerSystemRef/powerplant/mot/ctrl/cmd/parameter_selection ==
  inport-main_info_bus-1 : Inport
  select_main_info_bus : BusSelector  OutputSignals=apa_info_bus.powerplant_info_bus.mot.plant.mot_plant_spd_out_simu,apa_info_bus.powerplant_info_bus.mot.ctrl.dmd.mot_ctrl_trs_trq_simu,apa_info_bus.powerplant_info_bus.mot.ctrl.cstr.mot_ctrl_cstr_trq_max_pos_simu,apa_info_bus.powerplant_info_bus.mot.ctrl.cstr.mot_ctrl_cstr_trq_max_neg_simu
  outport-mot_plant_spd_out_simu-1 : Outport
  outport-mot_ctrl_trs_trq_simu-2 : Outport  Port=2
  outport-mot_ctrl_cstr_trq_max_pos_simu-3 : Outport  Port=3
  outport-mot_ctrl_cstr_trq_max_neg_simu-4 : Outport  Port=4
  wires:
  inport-main_info_bus-1/1 -> select_main_info_bus/1
  select_main_info_bus/1 -> outport-mot_plant_spd_out_simu-1/1  "<mot_plant_spd_out_simu>"
  select_main_info_bus/2 -> outport-mot_ctrl_trs_trq_simu-2/1  "<mot_ctrl_trs_trq_simu>"
  select_main_info_bus/3 -> outport-mot_ctrl_cstr_trq_max_pos_simu-3/1  "<mot_ctrl_cstr_trq_max_pos_simu>"
  select_main_info_bus/4 -> outport-mot_ctrl_cstr_trq_max_neg_simu-4/1  "<mot_ctrl_cstr_trq_max_neg_simu>"

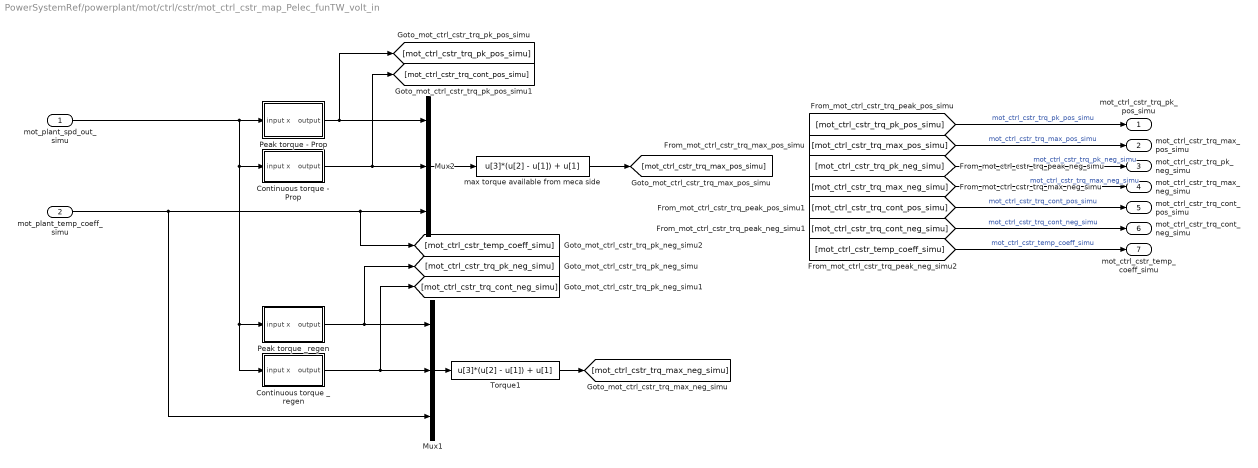
== system PowerSystemRef/powerplant/mot/ctrl/cstr/mot_ctrl_cstr_map_Pelec_funTW_volt_in ==
  mot_plant_spd_out_simu : Inport
  mot_plant_temp_coeff_simu : Inport  Port=2
  Continuous torque - Prop : Subsystem  mask{x=mot.plant.init.trq_pos_cont.idx1_spd, map=mot.plant.init.trq_pos_cont.map}
      mask Display: image(imread('map1D.jpg','jpeg'))
  Continuous torque _regen : Subsystem  mask{x=mot.plant.init.trq_neg_cont.idx1_spd, map=mot.plant.init.trq_neg_cont.map}
      mask Display: image(imread('map1D.jpg','jpeg'))
  Mux1 : Mux  Inputs=3
  Mux2 : Mux  Inputs=3
  Peak torque - Prop : Subsystem  mask{x=mot.plant.init.trq_pos_max.idx1_spd, map=mot.plant.init.trq_pos_max.map}
      mask Display: image(imread('map1D.jpg','jpeg'))
  Peak torque _regen : Subsystem  mask{x=mot.plant.init.trq_neg_max.idx1_spd, map=mot.plant.init.trq_neg_max.map}
      mask Display: image(imread('map1D.jpg','jpeg'))
  Torque1 : Fcn  Expr=u[3]*(u[2] - u[1]) + u[1]
  max torque available from meca side : Fcn  Expr=u[3]*(u[2] - u[1]) + u[1]
  mot_ctrl_cstr_trq_pk_pos_simu : Outport
  mot_ctrl_cstr_trq_max_pos_simu : Outport  Port=2
  mot_ctrl_cstr_trq_pk_neg_simu : Outport  Port=3
  mot_ctrl_cstr_trq_max_neg_simu : Outport  Port=4
  mot_ctrl_cstr_trq_cont_pos_simu : Outport  Port=5
  mot_ctrl_cstr_trq_cont_neg_simu : Outport  Port=6
  mot_ctrl_cstr_temp_coeff_simu : Outport  Port=7
  wires:
  [mot_ctrl_cstr_temp_coeff_simu] -> mot_ctrl_cstr_temp_coeff_simu/1  "mot_ctrl_cstr_temp_coeff_simu"
  [mot_ctrl_cstr_trq_cont_neg_simu] -> mot_ctrl_cstr_trq_cont_neg_simu/1  "mot_ctrl_cstr_trq_cont_neg_simu"
  [mot_ctrl_cstr_trq_cont_pos_simu] -> mot_ctrl_cstr_trq_cont_pos_simu/1  "mot_ctrl_cstr_trq_cont_pos_simu"
  [mot_ctrl_cstr_trq_pk_neg_simu] -> mot_ctrl_cstr_trq_pk_neg_simu/1  "mot_ctrl_cstr_trq_pk_neg_simu"
  [mot_ctrl_cstr_trq_max_neg_simu] -> mot_ctrl_cstr_trq_max_neg_simu/1  "mot_ctrl_cstr_trq_max_neg_simu"
  [mot_ctrl_cstr_trq_max_pos_simu] -> mot_ctrl_cstr_trq_max_pos_simu/1  "mot_ctrl_cstr_trq_max_pos_simu"
  [mot_ctrl_cstr_trq_pk_pos_simu] -> mot_ctrl_cstr_trq_pk_pos_simu/1  "mot_ctrl_cstr_trq_pk_pos_simu"
  mot_plant_spd_out_simu/1 -> Continuous torque _regen/1(input x), Peak torque _regen/1(input x), Continuous torque - Prop/1(input x), Peak torque - Prop/1(input x)
  Peak torque _regen/1(output) -> Mux1/1, [mot_ctrl_cstr_trq_pk_neg_simu]
  Peak torque - Prop/1(output) -> [mot_ctrl_cstr_trq_pk_pos_simu], Mux2/1
  mot_plant_temp_coeff_simu/1 -> [mot_ctrl_cstr_temp_coeff_simu], Mux2/3, Mux1/3
  Mux1/1 -> Torque1/1
  Continuous torque _regen/1(output) -> [mot_ctrl_cstr_trq_cont_neg_simu], Mux1/2
  Mux2/1 -> max torque available from meca side/1
  Continuous torque - Prop/1(output) -> [mot_ctrl_cstr_trq_cont_pos_simu], Mux2/2
  Torque1/1 -> [mot_ctrl_cstr_trq_max_neg_simu]
  max torque available from meca side/1 -> [mot_ctrl_cstr_trq_max_pos_simu]

== system PowerSystemRef/powerplant/mot/ctrl/cstr/parameter_out ==
  inport-mot_ctrl_cstr_trq_pk_pos_simu : Inport
  inport-mot_ctrl_cstr_trq_max_pos_simu : Inport  Port=2
  inport-mot_ctrl_cstr_trq_pk_neg_simu : Inport  Port=3
  inport-mot_ctrl_cstr_trq_max_neg_simu : Inport  Port=4
  inport-mot_ctrl_cstr_trq_cont_pos_simu : Inport  Port=5
  inport-mot_ctrl_cstr_trq_cont_neg_simu : Inport  Port=6
  inport-mot_ctrl_cstr_temp_coeff_simu : Inport  Port=7
  Ground_1 : Ground
  Toworkspace-mot_ctrl_cstr_temp_coeff_simu : ToWorkspace  VariableName=mot_ctrl_cstr_temp_coeff_simu  SampleTime=pxf_diagram_options.workspace_sample_time
      settings: Decimation=pxf_diagram_options.decimation
  Toworkspace-mot_ctrl_cstr_trq_cont_neg_simu : ToWorkspace  VariableName=mot_ctrl_cstr_trq_cont_neg_simu  SampleTime=pxf_diagram_options.workspace_sample_time
      settings: Decimation=pxf_diagram_options.decimation
  Toworkspace-mot_ctrl_cstr_trq_cont_pos_simu : ToWorkspace  VariableName=mot_ctrl_cstr_trq_cont_pos_simu  SampleTime=pxf_diagram_options.workspace_sample_time
      settings: Decimation=pxf_diagram_options.decimation
  Toworkspace-mot_ctrl_cstr_trq_max_neg_simu : ToWorkspace  VariableName=mot_ctrl_cstr_trq_max_neg_simu  SampleTime=pxf_diagram_options.workspace_sample_time
      settings: Decimation=pxf_diagram_options.decimation
  Toworkspace-mot_ctrl_cstr_trq_max_pos_simu : ToWorkspace  VariableName=mot_ctrl_cstr_trq_max_pos_simu  SampleTime=pxf_diagram_options.workspace_sample_time
      settings: Decimation=pxf_diagram_options.decimation
  Toworkspace-mot_ctrl_cstr_trq_pk_neg_simu : ToWorkspace  VariableName=mot_ctrl_cstr_trq_pk_neg_simu  SampleTime=pxf_diagram_options.workspace_sample_time
      settings: Decimation=pxf_diagram_options.decimation
  Toworkspace-mot_ctrl_cstr_trq_pk_pos_simu : ToWorkspace  VariableName=mot_ctrl_cstr_trq_pk_pos_simu  SampleTime=pxf_diagram_options.workspace_sample_time
      settings: Decimation=pxf_diagram_options.decimation
  create_system_info_bus : BusCreator  Inputs=2
  outport-system_info_bus : Outport
  outport-cstr_bus : Outport  Port=2
  wires:
  create_system_info_bus/1 -> outport-system_info_bus/1
  inport-mot_ctrl_cstr_trq_pk_pos_simu/1 -> Toworkspace-mot_ctrl_cstr_trq_pk_pos_simu/1
  inport-mot_ctrl_cstr_trq_max_pos_simu/1 -> create_system_info_bus/1, Toworkspace-mot_ctrl_cstr_trq_max_pos_simu/1  "mot_ctrl_cstr_trq_max_pos_simu"
  inport-mot_ctrl_cstr_trq_pk_neg_simu/1 -> Toworkspace-mot_ctrl_cstr_trq_pk_neg_simu/1
  inport-mot_ctrl_cstr_trq_max_neg_simu/1 -> create_system_info_bus/2, Toworkspace-mot_ctrl_cstr_trq_max_neg_simu/1  "mot_ctrl_cstr_trq_max_neg_simu"
  inport-mot_ctrl_cstr_trq_cont_pos_simu/1 -> Toworkspace-mot_ctrl_cstr_trq_cont_pos_simu/1
  inport-mot_ctrl_cstr_trq_cont_neg_simu/1 -> Toworkspace-mot_ctrl_cstr_trq_cont_neg_simu/1
  inport-mot_ctrl_cstr_temp_coeff_simu/1 -> Toworkspace-mot_ctrl_cstr_temp_coeff_simu/1
  Ground_1/1 -> outport-cstr_bus/1

== system PowerSystemRef/powerplant/mot/ctrl/cstr/parameter_selection ==
  inport-main_info_bus-1 : Inport
  select_main_info_bus : BusSelector  OutputSignals=apa_info_bus.powerplant_info_bus.mot.plant.mot_plant_spd_out_simu,apa_info_bus.powerplant_info_bus.mot.plant.mot_plant_temp_coeff_simu
  outport-mot_plant_spd_out_simu-1 : Outport
  outport-mot_plant_temp_coeff_simu-2 : Outport  Port=2
  wires:
  inport-main_info_bus-1/1 -> select_main_info_bus/1
  select_main_info_bus/1 -> outport-mot_plant_spd_out_simu-1/1  "<mot_plant_spd_out_simu>"
  select_main_info_bus/2 -> outport-mot_plant_temp_coeff_simu-2/1  "<mot_plant_temp_coeff_simu>"
